simulink model "FuzzyMobileRobotGuidance"  (R2023a)
settings: Solver=ode45  StartTime=0.0  StopTime=100  RelTol=1e-3  EnableMultiTasking=on
libraries: fl_lib x20, nesl_utility x8, vrlib x7, simulink x5
settings Model: PacingRate=1000  Creator=WB  LastModifiedBy=wb
settings SolverCC: AlgebraicLoopSolver=TrustRegion
settings DataIOCC: LimitDataPoints=on  SaveFormat=Array  SignalLoggingSaveFormat=ModelDataLogs  ReturnWorkspaceOutputs=off
settings OptimizationCC: ExpressionDepthLimit=2147483647  LifeSpan=inf
settings DebuggingCC: UnderspecifiedInitializationDetection=Classic  MergeDetectMultiDrivingBlocksExec=none  FcnCallInpInsideContextMsg=warning  UnconnectedInputMsg=warning  UnconnectedOutputMsg=warning  UnconnectedLineMsg=warning  AllowSymbolicDim=off  StateNameClashWarn=warning  SFUnexpectedBacktrackingDiag=warning  SFNoUnconditionalDefaultTransitionDiag=warning  SFExecutionAtInitializationDiag=none  ArithmeticOperatorsInVariantConditions=warning
settings HardwareCC: ProdBitPerPointer=32  ProdBitPerSizeT=32  ProdBitPerPtrDiffT=32  ProdLargestAtomicFloat=None  ProdIntDivRoundTo=Undefined  ProdEndianess=Unspecified  ProdWordSize=32  ProdHWDeviceType=32-bit Generic
settings ModelReferenceCC: EnableRefExpFcnMdlSchedulingChecks=on  PropagateSignalLabelsOutOfModel=off
settings SFSimCC: SimUseLocalCustomCode=off  CustomCodeUndefinedFunction=UseInterfaceOnly
settings RTWCC: RTWUseLocalCustomCode=off
settings CodeAppCC: StateflowObjectComments=on
settings GRTTargetCC: TargetLangStandard=C89/C90 (ANSI)  CombineOutputUpdateFcns=off  GRTInterface=on
settings ConfigComp: CovMetricSettings=dw  CovSaveCumulativeToWorkspaceVar=on  CovSaveSingleToWorkspaceVar=on  CovExternalEMLEnable=off
settings SimscapeCC: SimscapeNormalizeSystem=off

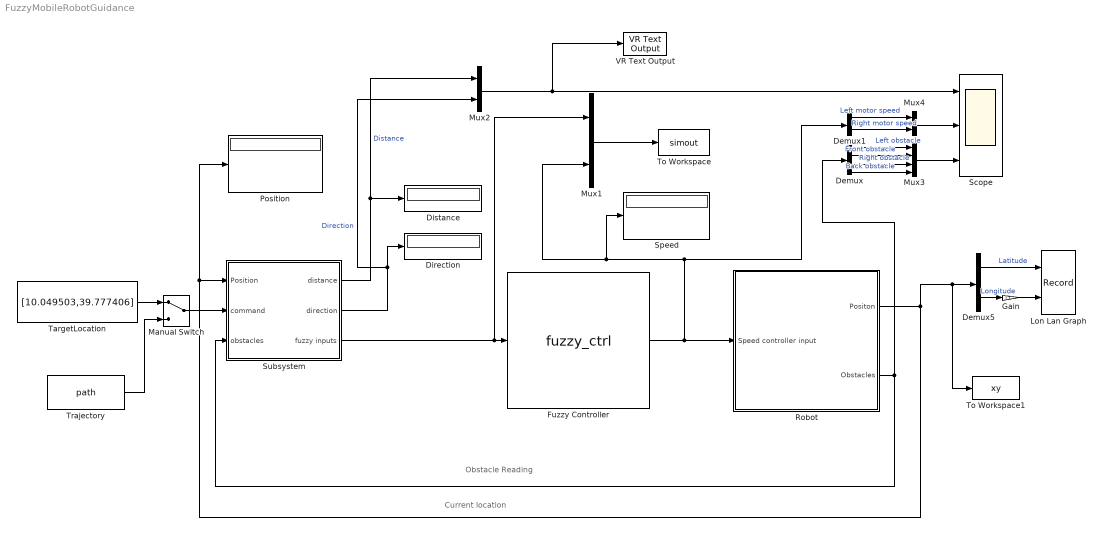
== system FuzzyMobileRobotGuidance ==
  note: Current location
  note: Obstacle Reading
  Demux : Demux
  Demux1 : Demux  Outputs=2
  Demux5 : Demux  Outputs=2
  Direction : Display
  Distance : Display
  Fuzzy Controller : S-Function  FunctionName=fuzzy_ctrl  SFunctionDeploymentMode=off  EnableBusSupport=off
  Gain : Gain  Gain=-1
  Lon Lan Graph : Record  FileSettingsInternal="{\"entries\":[{\"content\":{\"excelSettings\":{\"content\":{},\"type\":\"Streamout.ExcelSettings\"}},\"type\":\"Streamout.FileSettingStorage\",\"uuid\":\"\"}],\"packageUris\":[\"http:\\/\\/schema.mathworks.com\\/mf0\\/streamout_blocks\\/R2020a\"],\"version\":\"1.0\"}"  Layout=[1 1]  SignalsInternal="{\"entries\":[{\"content\":{\"signals\":[{\"content\":{\"blockPath\":[],\"dimensions\":[1],\"domain\":\"\",\"lineColor\":\"#a2142f\",\"plots\":[1],\"port\":1,\"sid\":[\"\"],\"signalID\":34161,\"signalName\":\"Latitude\"},\"type\":\"RecordBlkView.Signal\",\"uuid\":\"\"},{\"content\":{\"blockPath\":[],\"dimensions\":[1],\"domain\":\"\",\"lineColor\":\"#139fff\",\"plots\":[1],\"port\":2,\"sid\":[\"\"],\"signalID\":34165,\"signalName\":\"Gain\"},\"type\":\"RecordBlkView.Signal\",\"uuid\":\"\"}]},\"type\":\"RecordBlkView.InputSignals\",\"uuid\":\"\"}],\"packageUris\":[\"http:\\/\\/schema.mathworks.com\\/mf0\\/streamout_blocks\\/R2020a\"],\"version\":\"1.0\"}"  VisualizationBindings="{\"xyplotplugin\":{\"info\":[{\"series\":[{\"bindingParametersList\":[{\"parameter\":\"X-Axis\",\"signalID\":34161,\"signalName\":\"Latitude\"},{\"parameter\":\"Y-Axis\",\"signalID\":34165,\"signalName\":\"Gain\"}],\"seriesID\":15077}],\"subplotID\":1}]}}"  CompatibilityTag=XY  st=-1
  Manual Switch : ManualSwitch
  Mux1 : Mux  Inputs=2
  Mux2 : Mux  Inputs=2
  Mux3 : Mux
  Mux4 : Mux  Inputs=2
  Position : Display
  Robot : Subsystem
      mask Display: image(imread('robot.jpg'))
  Scope : Scope  NumInputPorts=3
  Speed : Display
  Subsystem : Subsystem
  TargetLocation : Constant  Tag=Target  Value=[10.049503,39.777406]  OutDataTypeStr=double
  To Workspace : ToWorkspace  VariableName=simout  SaveFormat=Structure With Time  SampleTime=-1
  To Workspace1 : ToWorkspace  VariableName=xy  SaveFormat=Timeseries  SampleTime=-1
  Trajectory : FromWorkspace  VariableName=path
  VR Text Output : vrlib/VR Text Output  VrmlFile=Robot.wrl  TxtNode=distance  FormatString=Distance: %7.2f m\nDirection: %7.2f deg\n  Ts=-1  ForceViewerOpen=off
  wires:
  Subsystem/3(fuzzy inputs) -> Fuzzy Controller/1, Mux1/1
  Robot/1(Positon) -> Position/1, Subsystem/1(Position), To Workspace1/1, Demux5/1
  Mux1/1 -> To Workspace/1
  Fuzzy Controller/1 -> Robot/1(Speed controller input), Demux1/1, Speed/1, Mux1/2
  Subsystem/2(direction) -> Direction/1, Mux2/2  "Direction"
  Subsystem/1(distance) -> Distance/1, Mux2/1  "Distance"
  Mux2/1 -> VR Text Output/1, Scope/1
  Robot/2(Obstacles) -> Subsystem/3(obstacles), Demux/1
  Demux/2 -> Mux3/2  "Front obstacle"
  Demux/4 -> Mux3/4  "Back obstacle"
  Demux/1 -> Mux3/1  "Left obstacle"
  Demux/3 -> Mux3/3  "Right obstacle"
  Mux3/1 -> Scope/3
  Demux1/1 -> Mux4/1  "Left motor speed"
  Demux1/2 -> Mux4/2  "Right motor speed"
  Mux4/1 -> Scope/2
  Demux5/1 -> Lon Lan Graph/1  "Latitude"
  Demux5/2 -> Gain/1  "Longitude"
  Gain/1 -> Lon Lan Graph/2
  TargetLocation/1 -> Manual Switch/1
  Manual Switch/1 -> Subsystem/2(command)
  Trajectory/1 -> Manual Switch/2

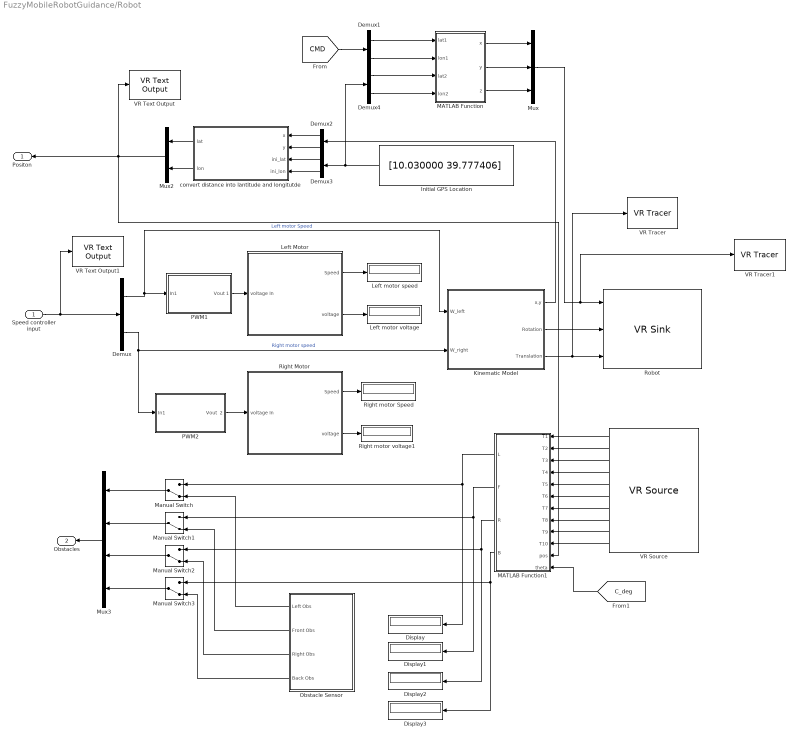
== system FuzzyMobileRobotGuidance/Robot ==
  Speed controller input : Inport
  Demux{,1..4} (5 alike) : Demux  Outputs=2
  Display{,1..3} (4 alike) : Display
  "Initial GPS Location " : Constant  Value=[10.030000 39.777406]
  Kinematic Model : Subsystem
  Left Motor : Subsystem
      mask Display: image(imread('maskIconDCMotor.png'))
  Left motor voltage : Display
  Left motor speed : Display
  MATLAB Function : MATLAB Function  TreatAsAtomicUnit=on
  MATLAB Function1 : MATLAB Function  TreatAsAtomicUnit=on
  Manual Switch{,1..3} (4 alike) : ManualSwitch  CurrentSetting=0
  Mux : Mux  Inputs=3
  Mux2 : Mux  Inputs=2
  Mux3 : Mux
  Obstacle Sensor : Subsystem
  PWM1 : Subsystem
  PWM2 : Subsystem
  Right Motor : Subsystem
      mask Display: image(imread('maskIconDCMotor.png'))
  Right motor voltage1 : Display
      settings: Format=bank
  Right motor Speed : Display
  Robot : vrlib/VR Sink  InstantiateOnLoad=on  SampleTime=0.1  ViewEnable=on  RemoteChange=off  RemoteView=on  FieldsWritten=Target.translation.3.1.1.double#Car.rotation.4.1.1.double#Car.translation.3.1.1.double  WorldFileName=Robot.wrl  AutoView=off  VideoDimensions=[]  AllowVariableSize=off
  VR Source : vrlib/VR Source  InstantiateOnLoad=on  SampleTime=0.1  ViewEnable=on  RemoteChange=off  RemoteView=on  FieldsRead=Obstacle.translation.1.3.1.double#palm_tree2.translation.1.3.1.double#Building3.translation.1.3.1.double#Building1.translation.1.3.1.double#palm_tree.translation.1.3.1.double#Tree3.translation.1.3.1.double#Tree4.translation.1.3.1.double#Building2.translation.1.3.1.double#Tree2.translation.1.3.1.double#Tree1.translation.1.3.1.double  WorldFileName=Robot.wrl  AutoView=off  VideoDimensions=[]  AllowVariableSize=off
  VR Text Output : vrlib/VR Text Output  VrmlFile=Robot.wrl  TxtNode=display  FormatString=Latitude: %7.6f deg\nLongitude: %7.6f deg\n  Ts=-1  ForceViewerOpen=off
  VR Text Output1 : vrlib/VR Text Output  VrmlFile=Robot.wrl  TxtNode=Speed  FormatString=Left Speed: %7.2f rpm\nRight Speed: %7.2f rpm\n  Ts=-1  ForceViewerOpen=off
  VR Tracer : vrlib/VR Tracer  VrmlFile=Robot.wrl  MarkerName=None  UseLines=on  UseTriads=on  MarkerScale=[1 1 1]  MarkerColorSelection=Selected from color list  MarkerColor=blue  rgbval=[1 0 0]  Ts=0.5  ForceViewerOpen=off  ConnectPlane=off  PlaneCoeff=[0 1 0 0]  ConnectPoint=None  PointCoord=[0 0 0]
  VR Tracer1 : vrlib/VR Tracer  VrmlFile=Robot.wrl  MarkerName=None  UseLines=on  UseTriads=on  MarkerScale=[1 1 1]  MarkerColorSelection=Selected from color list  MarkerColor=red  rgbval=[1 0 0]  Ts=0.5  ForceViewerOpen=off  ConnectPlane=off  PlaneCoeff=[0 1 0 0]  ConnectPoint=None  PointCoord=[0 0 0]
  convert distance into lantitude and longitutde : MATLAB Function  TreatAsAtomicUnit=on
  Positon : Outport
  Obstacles : Outport  Port=2
  wires:
  "Initial GPS Location "/1 -> Demux4/1, Demux3/1
  convert distance into lantitude and longitutde/2(lon) -> Mux2/2
  convert distance into lantitude and longitutde/1(lat) -> Mux2/1
  Demux3/2 -> convert distance into lantitude and longitutde/4(ini_lon)
  Demux3/1 -> convert distance into lantitude and longitutde/3(ini_lat)
  Demux2/2 -> convert distance into lantitude and longitutde/2(y)
  Demux2/1 -> convert distance into lantitude and longitutde/1(x)
  Kinematic Model/3(Translation) -> VR Tracer/1, Robot/3
  Demux/2 -> PWM2/1(In1), Kinematic Model/2(W_right)  "Right motor speed"
  Demux/1 -> PWM1/1(In1), Kinematic Model/1(W_left)  "Left motor Speed"
  Right Motor/2(voltage) -> Right motor voltage1/1
  Right Motor/1(Speed) -> Right motor Speed/1
  Left Motor/2(voltage) -> Left motor voltage/1
  Left Motor/1(Speed) -> Left motor speed/1
  Speed controller input/1 -> Demux/1, VR Text Output1/1
  Mux2/1 -> Positon/1, MATLAB Function1/11(pos), VR Text Output/1
  Mux3/1 -> Obstacles/1
  Kinematic Model/1(x,y) -> Demux2/1
  PWM1/1(Vout 1) -> Left Motor/1(voltage In)
  PWM2/1(Vout  2) -> Right Motor/1(voltage In)
  Kinematic Model/2(Rotation) -> Robot/2
  [CMD] -> Demux1/1
  Demux1/2 -> MATLAB Function/2(lon1)
  Demux1/1 -> MATLAB Function/1(lat1)
  Demux4/1 -> MATLAB Function/3(lat2)
  Demux4/2 -> MATLAB Function/4(lon2)
  MATLAB Function/2(y) -> Mux/2
  MATLAB Function/1(x) -> Mux/1
  MATLAB Function/3(z) -> Mux/3
  Mux/1 -> VR Tracer1/1, Robot/1
  [C_deg] -> MATLAB Function1/12(theta)
  VR Source/1 -> MATLAB Function1/1(T1)
  VR Source/2 -> MATLAB Function1/2(T2)
  VR Source/3 -> MATLAB Function1/3(T3)
  VR Source/4 -> MATLAB Function1/4(T4)
  VR Source/5 -> MATLAB Function1/5(T5)
  VR Source/6 -> MATLAB Function1/6(T6)
  VR Source/7 -> MATLAB Function1/7(T7)
  VR Source/8 -> MATLAB Function1/8(T8)
  VR Source/9 -> MATLAB Function1/9(T9)
  VR Source/10 -> MATLAB Function1/10(T10)
  MATLAB Function1/1(L) -> Manual Switch/1, Display/1
  MATLAB Function1/2(F) -> Manual Switch1/1, Display1/1
  MATLAB Function1/3(R) -> Manual Switch2/1, Display2/1
  MATLAB Function1/4(B) -> Manual Switch3/1, Display3/1
  Obstacle Sensor/1(Left Obs) -> Manual Switch/2
  Obstacle Sensor/2(Front Obs) -> Manual Switch1/2
  Obstacle Sensor/3(Right Obs) -> Manual Switch2/2
  Obstacle Sensor/4(Back Obs) -> Manual Switch3/2
  Manual Switch/1 -> Mux3/1
  Manual Switch1/1 -> Mux3/2
  Manual Switch2/1 -> Mux3/3
  Manual Switch3/1 -> Mux3/4

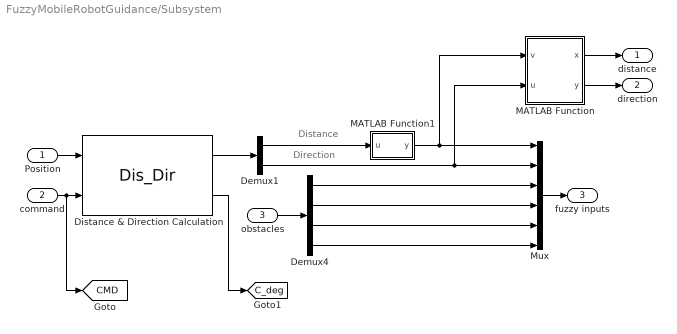
== system FuzzyMobileRobotGuidance/Subsystem ==
  note: Distance
  note: Direction
  Position : Inport
  command : Inport  Port=2
  obstacles : Inport  Port=3
  Demux1 : Demux  Outputs=2
  Demux4 : Demux
  Distance & Direction Calculation : S-Function  FunctionName=Dis_Dir  SFunctionDeploymentMode=off  EnableBusSupport=off
  MATLAB Function : MATLAB Function  TreatAsAtomicUnit=on
  MATLAB Function1 : MATLAB Function  TreatAsAtomicUnit=on
  Mux : Mux  Inputs=6
  distance : Outport
  direction : Outport  Port=2
  fuzzy inputs : Outport  Port=3
  tag scope: CMD=global, C_deg=global
  wires:
  Demux1/1 -> MATLAB Function1/1(u)
  Demux1/2 -> MATLAB Function/2(u), Mux/2
  Distance & Direction Calculation/1 -> Demux1/1
  Demux4/1 -> Mux/3
  Demux4/2 -> Mux/4
  Demux4/3 -> Mux/5
  Demux4/4 -> Mux/6
  Position/1 -> Distance & Direction Calculation/1
  command/1 -> [CMD], Distance & Direction Calculation/2
  Mux/1 -> fuzzy inputs/1
  obstacles/1 -> Demux4/1
  MATLAB Function/2(y) -> direction/1
  Distance & Direction Calculation/2 -> [C_deg]
  MATLAB Function/1(x) -> distance/1
  MATLAB Function1/1(y) -> MATLAB Function/1(v), Mux/1

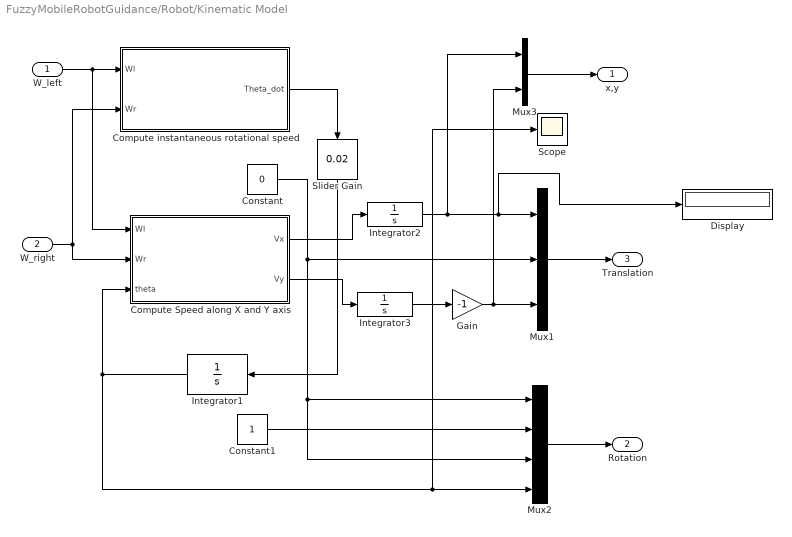
== system FuzzyMobileRobotGuidance/Robot/Kinematic Model ==
  W_left : Inport
  W_right : Inport  Port=2
  Compute Speed along X and Y axis : MATLAB Function  TreatAsAtomicUnit=on
  Compute instantaneous rotational speed : MATLAB Function  TreatAsAtomicUnit=on
  Constant : Constant  Value=0
  Constant1 : Constant
  Display : Display
  Gain : Gain  Gain=-1
  Integrator1 : Integrator
  Integrator2 : Integrator
  Integrator3 : Integrator
  Mux1 : Mux  Inputs=3
  Mux2 : Mux
  Mux3 : Mux  Inputs=2
  Scope : Scope
  Slider Gain : simulink/Math Operations/Slider Gain  gain=0.02  low=0  high=2
  x,y : Outport
  Rotation : Outport  Port=2
  Translation : Outport  Port=3
  wires:
  Compute instantaneous rotational speed/1(Theta_dot) -> Slider Gain/1
  Integrator1/1 -> Compute Speed along X and Y axis/3(theta), Mux2/4, Scope/1
  Compute Speed along X and Y axis/1(Vx) -> Integrator2/1
  Compute Speed along X and Y axis/2(Vy) -> Integrator3/1
  Integrator2/1 -> Display/1, Mux1/1, Mux3/1
  Integrator3/1 -> Gain/1
  Constant/1 -> Mux1/2, Mux2/3, Mux2/1
  Constant1/1 -> Mux2/2
  W_left/1 -> Compute instantaneous rotational speed/1(Wl), Compute Speed along X and Y axis/1(Wl)
  W_right/1 -> Compute instantaneous rotational speed/2(Wr), Compute Speed along X and Y axis/2(Wr)
  Mux1/1 -> Translation/1
  Mux2/1 -> Rotation/1
  Slider Gain/1 -> Integrator1/1
  Gain/1 -> Mux3/2, Mux1/3
  Mux3/1 -> x,y/1

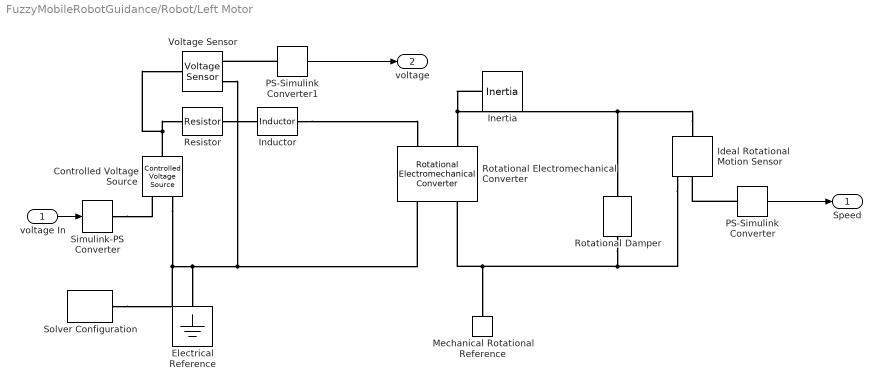
== system FuzzyMobileRobotGuidance/Robot/Left Motor ==
  voltage In : Inport
  Controlled Voltage Source : fl_lib/Electrical/Electrical Sources/Controlled Voltage Source
  Electrical Reference : fl_lib/Electrical/Electrical Elements/Electrical Reference
  Ideal Rotational Motion Sensor : fl_lib/Mechanical/Mechanical Sensors/Ideal Rotational Motion Sensor  reference=foundation.enum.MeasurementReference.difference  acceleration_port=false  velocity_port=true  position_port=true  wrap_angle=false  offset=0 rad
  Inductor : fl_lib/Electrical/Electrical Elements/Inductor  l=0.5 H  r=0 Ohm  g=1e-9 1/Ohm  i_specify=off  i_priority=None  i=0 A  i_nominal_specify=off  i_nominal_unit=A  i_nominal_value=1  v_specify=off  v_priority=None  v=0 V  v_nominal_specify=off  v_nominal_unit=V  v_nominal_value=1  i_L_specify=on  i_L_priority=High  i_L=0 A  i_L_nominal_specify=off  i_L_nominal_unit=A  i_L_nominal_value=1
  Inertia : fl_lib/Mechanical/Rotational Elements/Inertia  inertia=0.01 kg*m^2  num_ports=foundation.enum.numPorts2.one  w_specify=on  w_priority=High  w=0 rad/s  w_nominal_specify=off  w_nominal_unit=rad/s  w_nominal_value=1  t_specify=off  t_priority=None  t=0 N*m  t_nominal_specify=off  t_nominal_unit=N*m  t_nominal_value=1
  Mechanical Rotational Reference : fl_lib/Mechanical/Rotational Elements/Mechanical Rotational Reference
  PS-Simulink Converter : nesl_utility/PS-Simulink Converter  PhysicalDomain=network_engine_domain  SubClassName=ps_output  LeftPortType=input  RightPortType=output  PseudoPeriodic=off  Frequencies=[]  VectorFormat=1-D array  Unit=1  AffineConversion=off
  PS-Simulink Converter1 : nesl_utility/PS-Simulink Converter  PhysicalDomain=network_engine_domain  SubClassName=ps_output  LeftPortType=input  RightPortType=output  PseudoPeriodic=off  Frequencies=[]  VectorFormat=1-D array  Unit=1  AffineConversion=off
  Resistor : fl_lib/Electrical/Electrical Elements/Resistor  R=1 Ohm  i_specify=off  i_priority=None  i=0 A  i_nominal_specify=off  i_nominal_unit=A  i_nominal_value=1  v_specify=off  v_priority=None  v=0 V  v_nominal_specify=off  v_nominal_unit=V  v_nominal_value=1
  Rotational Electromechanical Converter : fl_lib/Electrical/Electrical Elements/Rotational Electromechanical Converter  K=0.1 V/(rad/s)  i_specify=off  i_priority=None  i=0 A  i_nominal_specify=off  i_nominal_unit=A  i_nominal_value=1  v_specify=off  v_priority=None  v=0 V  v_nominal_specify=off  v_nominal_unit=V  v_nominal_value=1  t_specify=off  t_priority=None  t=0 N*m  t_nominal_specify=off  t_nominal_unit=N*m  t_nominal_value=1  w_specify=off  w_priority=None  w=0 rad/s  w_nominal_specify=off  w_nominal_unit=rad/s  w_nominal_value=1
  Rotational Damper : fl_lib/Mechanical/Rotational Elements/Rotational Damper  D=0.001 N*m/(rad/s)  w_specify=off  w_priority=None  w=0 rad/s  w_nominal_specify=off  w_nominal_unit=rad/s  w_nominal_value=1  t_specify=off  t_priority=None  t=0 N*m  t_nominal_specify=off  t_nominal_unit=N*m  t_nominal_value=1
  Simulink-PS Converter : nesl_utility/Simulink-PS Converter  PhysicalDomain=network_engine_domain  SubClassName=ps_input  LeftPortType=input  RightPortType=output  PseudoPeriodic=off  Frequencies=[]  NoiseDistribution=none  NoiseParameters=[]  Unit=1  AffineConversion=off  FilteringAndDerivatives=zero  SimscapeFilterOrder=1  InputFilterTimeConstant=.001  UdotUserProvided=0
  Solver Configuration : nesl_utility/Solver Configuration  PhysicalDomain=network_engine_domain  SubClassName=solver  LeftPortType=input  RightPortType=generic  Tones=[]  Harmonics=[]  SimulateNoise=off  Profile=off  UseLocalSampling=off  EnableSwitchedLinearOptims=on  FrequencyDomain=off  UseCCode=off  RelTol=0.001  AbsTol=1e-06  MinStep=1e-09  ToWorkspace=off  RevertToSquareIcSolve=off  NumHomotopyIterations=100  PhasorMode=off  PhasorModeNumHarmonics=1  ConsistencySolver=NEWTON_FTOL  IndexReductionMethod=DerivativeReplacement  DoDC=off  ResidualTolerance=1e-9  ConsistencyTolSource=GLOBAL  ConsistencyAbsTol=0.001  ConsistencyRelTol=0.001  ConsistencyTolFactor=0.001  UseLocalSolver=off  LocalSolverChoice=NE_BACKWARD_EULER_ADVANCER  ResolveIndetEquations=on  FunctionEvalNumThread=1  LocalSolverSampleTime=.001  DoFixedCost=off  MaxNonlinIter=3  MaxModeIter=2  ComputeImpulses=off  ImpulseIterations=2  LinearAlgebra=Sparse  LinearAlgebraNumThread=0  EquationFormulation=NE_TIME_EF  DelaysMemoryBudget=1024  AutomaticFiltering=on  FilteringTimeConstant=0.001  PartitionStorageMethod=AS_NEEDED  PartitionMemoryBudget=1024  PartitionMethod=FAST
  Voltage Sensor : fl_lib/Electrical/Electrical Sensors/Voltage Sensor
  Speed : Outport
  voltage : Outport  Port=2
  wires:
  voltage In/1 -> Simulink-PS Converter/1
  PS-Simulink Converter/1 -> Speed/1
  PS-Simulink Converter1/1 -> voltage/1
  connections:
  Controlled Voltage Source/LConn1 -- Resistor/LConn1 -- Voltage Sensor/LConn1
  Simulink-PS Converter/RConn1 -- Controlled Voltage Source/RConn1
  Controlled Voltage Source/RConn2 -- Electrical Reference/LConn1 -- Rotational Electromechanical Converter/RConn1 -- Voltage Sensor/RConn2 -- Solver Configuration/RConn1
  Inductor/RConn1 -- Rotational Electromechanical Converter/LConn1
  Ideal Rotational Motion Sensor/LConn1 -- Inertia/LConn1 -- Rotational Electromechanical Converter/LConn2 -- Rotational Damper/LConn1
  Ideal Rotational Motion Sensor/RConn1 -- Rotational Damper/RConn1 -- Rotational Electromechanical Converter/RConn2 -- Mechanical Rotational Reference/LConn1
  Resistor/RConn1 -- Inductor/LConn1
  PS-Simulink Converter1/LConn1 -- Voltage Sensor/RConn1
  PS-Simulink Converter/LConn1 -- Ideal Rotational Motion Sensor/RConn2

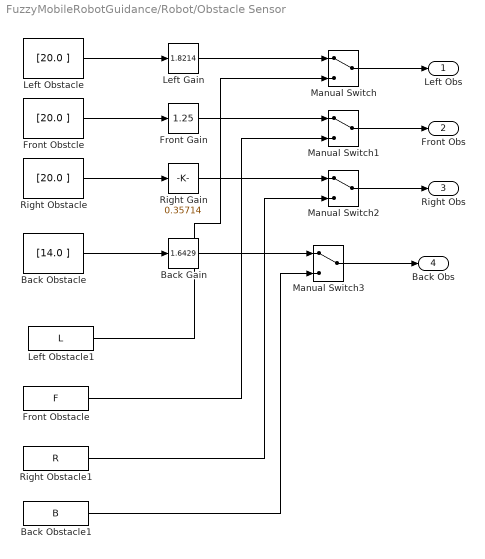
== system FuzzyMobileRobotGuidance/Robot/Obstacle Sensor ==
  Back Gain : simulink/Math Operations/Slider Gain  gain=1.6429  low=0  high=10
  Back Obstacle : Constant  Value=[14.0 ]
  Back Obstacle1 : FromWorkspace  VariableName=B
  Front Gain : simulink/Math Operations/Slider Gain  gain=1.25  low=0  high=10
  Front Obstacle : FromWorkspace  VariableName=F
  Front Obstcle : Constant  Value=[20.0 ]
  Left Gain : simulink/Math Operations/Slider Gain  gain=1.8214  low=0  high=10
  Left Obstacle : Constant  Value=[20.0 ]
  Left Obstacle1 : FromWorkspace  VariableName=L
  Manual Switch{,1..3} (4 alike) : ManualSwitch
  Right Gain : simulink/Math Operations/Slider Gain  gain=0.35714  low=0  high=10
  Right Obstacle : Constant  Value=[20.0 ]
  Right Obstacle1 : FromWorkspace  VariableName=R
  Left Obs : Outport
  Front Obs : Outport  Port=2
  Right Obs : Outport  Port=3
  Back Obs : Outport  Port=4
  wires:
  Left Obstacle/1 -> Left Gain/1
  Front Obstcle/1 -> Front Gain/1
  Right Obstacle/1 -> Right Gain/1
  Back Obstacle/1 -> Back Gain/1
  Left Obstacle1/1 -> Manual Switch/2
  Front Obstacle/1 -> Manual Switch1/2
  Right Obstacle1/1 -> Manual Switch2/2
  Back Obstacle1/1 -> Manual Switch3/2
  Left Gain/1 -> Manual Switch/1
  Manual Switch/1 -> Left Obs/1
  Front Gain/1 -> Manual Switch1/1
  Manual Switch1/1 -> Front Obs/1
  Right Gain/1 -> Manual Switch2/1
  Manual Switch2/1 -> Right Obs/1
  Back Gain/1 -> Manual Switch3/1
  Manual Switch3/1 -> Back Obs/1

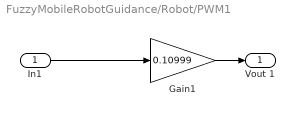
== system FuzzyMobileRobotGuidance/Robot/PWM1 ==
  In1 : Inport
  Gain1 : Gain  Gain=0.10999
  Vout 1 : Outport
  wires:
  Gain1/1 -> Vout 1/1
  In1/1 -> Gain1/1

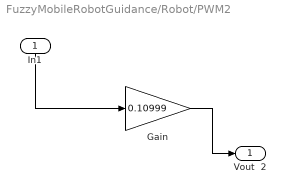
== system FuzzyMobileRobotGuidance/Robot/PWM2 ==
  In1 : Inport
  Gain : Gain  Gain=0.10999
  Vout  2 : Outport
  wires:
  Gain/1 -> Vout  2/1
  In1/1 -> Gain/1

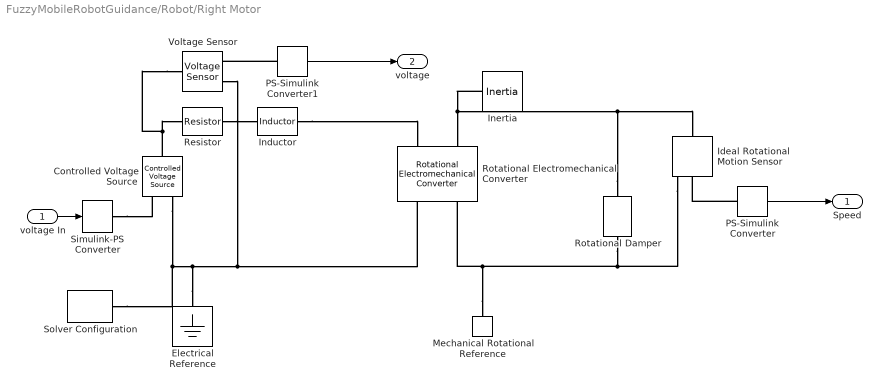
== system FuzzyMobileRobotGuidance/Robot/Right Motor ==
  voltage In : Inport
  Controlled Voltage Source : fl_lib/Electrical/Electrical Sources/Controlled Voltage Source
  Electrical Reference : fl_lib/Electrical/Electrical Elements/Electrical Reference
  Ideal Rotational Motion Sensor : fl_lib/Mechanical/Mechanical Sensors/Ideal Rotational Motion Sensor  reference=foundation.enum.MeasurementReference.difference  acceleration_port=false  velocity_port=true  position_port=true  wrap_angle=false  offset=0 rad
  Inductor : fl_lib/Electrical/Electrical Elements/Inductor  l=0.5 H  r=0 Ohm  g=1e-9 1/Ohm  i_specify=off  i_priority=None  i=0 A  i_nominal_specify=off  i_nominal_unit=A  i_nominal_value=1  v_specify=off  v_priority=None  v=0 V  v_nominal_specify=off  v_nominal_unit=V  v_nominal_value=1  i_L_specify=on  i_L_priority=High  i_L=0 A  i_L_nominal_specify=off  i_L_nominal_unit=A  i_L_nominal_value=1
  Inertia : fl_lib/Mechanical/Rotational Elements/Inertia  inertia=0.01 kg*m^2  num_ports=foundation.enum.numPorts2.one  w_specify=on  w_priority=High  w=0 rad/s  w_nominal_specify=off  w_nominal_unit=rad/s  w_nominal_value=1  t_specify=off  t_priority=None  t=0 N*m  t_nominal_specify=off  t_nominal_unit=N*m  t_nominal_value=1
  Mechanical Rotational Reference : fl_lib/Mechanical/Rotational Elements/Mechanical Rotational Reference
  PS-Simulink Converter : nesl_utility/PS-Simulink Converter  PhysicalDomain=network_engine_domain  SubClassName=ps_output  LeftPortType=input  RightPortType=output  PseudoPeriodic=off  Frequencies=[]  VectorFormat=1-D array  Unit=1  AffineConversion=off
  PS-Simulink Converter1 : nesl_utility/PS-Simulink Converter  PhysicalDomain=network_engine_domain  SubClassName=ps_output  LeftPortType=input  RightPortType=output  PseudoPeriodic=off  Frequencies=[]  VectorFormat=1-D array  Unit=1  AffineConversion=off
  Resistor : fl_lib/Electrical/Electrical Elements/Resistor  R=1 Ohm  i_specify=off  i_priority=None  i=0 A  i_nominal_specify=off  i_nominal_unit=A  i_nominal_value=1  v_specify=off  v_priority=None  v=0 V  v_nominal_specify=off  v_nominal_unit=V  v_nominal_value=1
  Rotational Electromechanical Converter : fl_lib/Electrical/Electrical Elements/Rotational Electromechanical Converter  K=0.1 V/(rad/s)  i_specify=off  i_priority=None  i=0 A  i_nominal_specify=off  i_nominal_unit=A  i_nominal_value=1  v_specify=off  v_priority=None  v=0 V  v_nominal_specify=off  v_nominal_unit=V  v_nominal_value=1  t_specify=off  t_priority=None  t=0 N*m  t_nominal_specify=off  t_nominal_unit=N*m  t_nominal_value=1  w_specify=off  w_priority=None  w=0 rad/s  w_nominal_specify=off  w_nominal_unit=rad/s  w_nominal_value=1
  Rotational Damper : fl_lib/Mechanical/Rotational Elements/Rotational Damper  D=0.001 N*m/(rad/s)  w_specify=off  w_priority=None  w=0 rad/s  w_nominal_specify=off  w_nominal_unit=rad/s  w_nominal_value=1  t_specify=off  t_priority=None  t=0 N*m  t_nominal_specify=off  t_nominal_unit=N*m  t_nominal_value=1
  Simulink-PS Converter : nesl_utility/Simulink-PS Converter  PhysicalDomain=network_engine_domain  SubClassName=ps_input  LeftPortType=input  RightPortType=output  PseudoPeriodic=off  Frequencies=[]  NoiseDistribution=none  NoiseParameters=[]  Unit=1  AffineConversion=off  FilteringAndDerivatives=zero  SimscapeFilterOrder=1  InputFilterTimeConstant=.001  UdotUserProvided=0
  Solver Configuration : nesl_utility/Solver Configuration  PhysicalDomain=network_engine_domain  SubClassName=solver  LeftPortType=input  RightPortType=generic  Tones=[]  Harmonics=[]  SimulateNoise=off  Profile=off  UseLocalSampling=off  EnableSwitchedLinearOptims=on  FrequencyDomain=off  UseCCode=off  RelTol=0.001  AbsTol=1e-06  MinStep=1e-09  ToWorkspace=off  RevertToSquareIcSolve=off  NumHomotopyIterations=100  PhasorMode=off  PhasorModeNumHarmonics=1  ConsistencySolver=NEWTON_FTOL  IndexReductionMethod=DerivativeReplacement  DoDC=off  ResidualTolerance=1e-9  ConsistencyTolSource=GLOBAL  ConsistencyAbsTol=0.001  ConsistencyRelTol=0.001  ConsistencyTolFactor=0.001  UseLocalSolver=off  LocalSolverChoice=NE_BACKWARD_EULER_ADVANCER  ResolveIndetEquations=on  FunctionEvalNumThread=1  LocalSolverSampleTime=.001  DoFixedCost=off  MaxNonlinIter=3  MaxModeIter=2  ComputeImpulses=off  ImpulseIterations=2  LinearAlgebra=Sparse  LinearAlgebraNumThread=0  EquationFormulation=NE_TIME_EF  DelaysMemoryBudget=1024  AutomaticFiltering=on  FilteringTimeConstant=0.001  PartitionStorageMethod=AS_NEEDED  PartitionMemoryBudget=1024  PartitionMethod=FAST
  Voltage Sensor : fl_lib/Electrical/Electrical Sensors/Voltage Sensor
  Speed : Outport
  voltage : Outport  Port=2
  wires:
  PS-Simulink Converter1/1 -> voltage/1
  PS-Simulink Converter/1 -> Speed/1
  voltage In/1 -> Simulink-PS Converter/1
  connections:
  PS-Simulink Converter/LConn1 -- Ideal Rotational Motion Sensor/RConn2
  PS-Simulink Converter1/LConn1 -- Voltage Sensor/RConn1
  Resistor/RConn1 -- Inductor/LConn1
  Mechanical Rotational Reference/LConn1 -- Rotational Electromechanical Converter/RConn2 -- Ideal Rotational Motion Sensor/RConn1 -- Rotational Damper/RConn1
  Rotational Damper/LConn1 -- Ideal Rotational Motion Sensor/LConn1 -- Rotational Electromechanical Converter/LConn2 -- Inertia/LConn1
  Inductor/RConn1 -- Rotational Electromechanical Converter/LConn1
  Electrical Reference/LConn1 -- Solver Configuration/RConn1 -- Controlled Voltage Source/RConn2 -- Voltage Sensor/RConn2 -- Rotational Electromechanical Converter/RConn1
  Simulink-PS Converter/RConn1 -- Controlled Voltage Source/RConn1
  Voltage Sensor/LConn1 -- Resistor/LConn1 -- Controlled Voltage Source/LConn1

== matlab function FuzzyMobileRobotGuidance/Robot/Kinematic Model/Compute instantaneous rotational speed ==
  data: Wl input; Wr input; Theta_dot output
function Theta_dot = fcn(Wl,Wr)
%#eml
l=0.65;%0.65
r=0.25;%0.25
Theta_dot=((Wr*r-Wl*r)/(2*l));%*(2*pi)/60;
end

== matlab function FuzzyMobileRobotGuidance/Robot/Kinematic Model/Compute Speed along X and Y axis ==
  data: Wl input; Wr input; Vx output; Vy output; theta input
function [Vx,Vy] = fcn(Wl,Wr,theta)
%#eml
%l=65.0;
r=0.25;%0.25
Vx  = ((Wr*r*cos(theta)+Wl*r*cos(theta))/2);%*(2*pi)/60;
Vy  = ((Wr*r*sin(theta)+Wl*r*sin(theta))/2);%*(2*pi)/60;
end

== matlab function FuzzyMobileRobotGuidance/Robot/convert distance into lantitude and longitutde ==
  data: x input; y input; lat output; lon output; ini_lat input; ini_lon input
function [lat,lon] = fcn(x,y,ini_lat,ini_lon)
%earth radius
r=6371000.00;
la=(360/(2*pi*r))*x;
lo=(360/(2*pi*r))*y;
lat=ini_lat+la;
lon=ini_lon+lo;
end

== matlab function FuzzyMobileRobotGuidance/Subsystem/MATLAB Function ==
  data: v input; x output; u input; y output
function[x, y] = fcn(v,u)
%#codegen
x=v/20;
if(u>180)
    y=u-360;
else
    y = u;
end
end

== matlab function FuzzyMobileRobotGuidance/Robot/MATLAB Function ==
  data: x output; lat1 input; y output; lon1 input; z output; lat2 input; lon2 input
function [x,y,z] = fcn(lat1,lon1,lat2,lon2)
%#codegen
r=6371000.00;
lat=lat1-lat2;
lon=lon1-lon2;
x=lat*((2*pi*r)/360);
z=lon*((2*pi*r)/360);
y=0;

== matlab function FuzzyMobileRobotGuidance/Robot/MATLAB Function1 ==
  data: L output; F output; R output; T1 input; T2 input; B output; T3 input; T4 input; T5 input; T6 input; T7 input; T8 input; T9 input; T10 input; pos input; theta input
function [L,F,R,B]=fnc(T1,T2,T3,T4,T5,T6,T7,T8,T9,T10,pos,theta)
%#codegen
L=100;
F=100;
R=100;
B=100;
r=6371000.00;
A=[T1(1),T1(2),T1(3);T2(1),T2(2),T2(3);...
    T3(1),T3(2),T3(3);T4(1),T4(2),T4(3);...
    T5(1),T5(2),T5(3);T6(1),T6(2),T6(3);...
    T7(1),T7(2),T7(3);T8(1),T8(2),T8(3);...
    T9(1),T9(2),T9(3);T10(1),T10(2),T10(3)];
for k=1:1:10
x=A(k,1);
y=A(k,3);
la0=pos(1);
lo0=pos(2);
la1=((360/(2*pi*r))*x)+10.030000 ;
lo1=((360/(2*pi*r))*y)+39.777406;
dist=(Distance(la0, lo0, la1, lo1))/50;
dir=direction(la0, lo0, la1, lo1);

byrig=(theta-dir);

    if(byrig<0)
      ang=byrig+360;
    else
      ang=byrig; 
    end
    if(((ang>=0 && ang < 10 )|| (ang <=360 && ang> 350))&& dist<F)
        F=dist;
    end
    if((ang>=20 && ang<100)&& dist<L)
        L=dist;
    end
  
    if((ang>=160 && ang<200)&& dist<B)
         B=dist;
    end
    if((ang>=260 && ang<350)&& dist<R)
        R=dist;
    end
end
end

== matlab function FuzzyMobileRobotGuidance/Subsystem/MATLAB Function1 ==
  data: u input; y output
function y = fcn(u)
%#codegen

if(u>2)
    y=u;
else
    y=0;
end
end
